simulink model "adcddcxaui_100"  (Simulink 6.2)
settings: Solver=ode45  StartTime=0.0  StopTime=1000  RelTol=1e-3
undefined symbols (not defined in the file): BitWidth
libraries: xbsIndex_r3 x358, casper_library x26, xps_library x12
(part 1 of 4)
settings Model: LastModifiedBy=lspitler
settings DebuggingCC: SolverPrmCheckMsg=warning

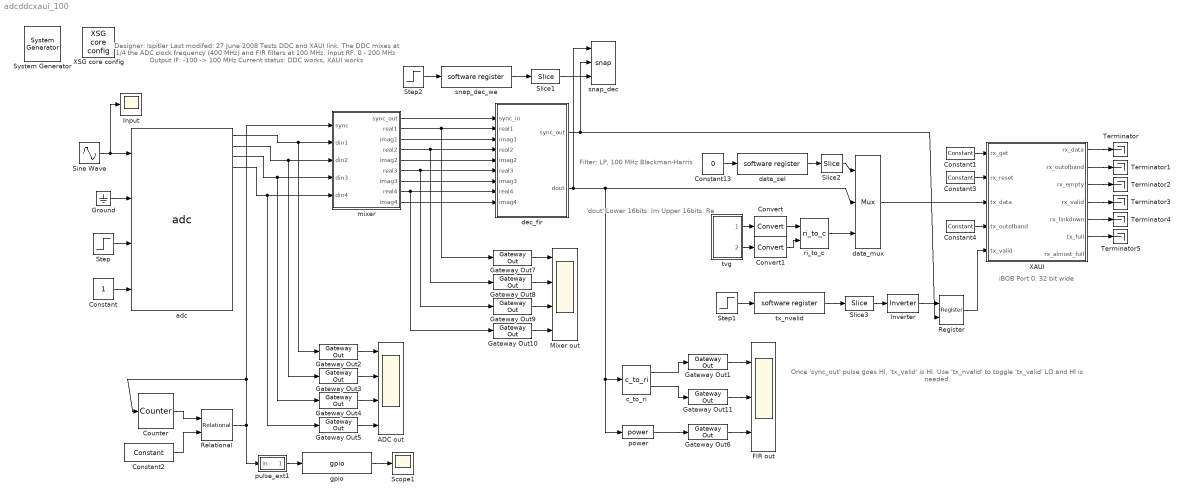
== system adcddcxaui_100 ==
  note: Designer: lspitler
      | Last modifed: 27 June 2008
      | Tests DDC and XAUI link.
      | The DDC mixes at 1/4 the ADC clock frequency (400 MHz)
      | and FIR filters at 100 MHz.
      | Input RF:  0 - 200 MHz
      | Output IF: -100 -> 100 MHz
      | Current status: DDC works, XAUI works
  note: Filter:
      | LP, 100 MHz Blackman-Harris
  note: 'dout'
      | Lower 16bits: Im
      | Upper 16bits: Re
  note: iBOB Port 0: 32 bit wide
  note: Once 'sync_out' pulse goes
      | HI, 'tx_valid' is HI.
      | Use 'tx_nvalid' to toggle
      | 'tx_valid' LO and HI is needed.
  " System Generator" : xbsIndex_r3/ System Generator  Tag=genX  xilinxfamily=Virtex2P  part=xc2vp50  speed=-7  package=ff1152  synthesis_tool=XST  directory=./adcddcxaui/sysgen  testbench=off  simulink_period=1  sysclk_period=5  incr_netlist=off  trim_vbits=Everywhere in SubSystem  dbl_ovrd=According to Block Masks  core_generation=According to Block Masks  run_coregen=off  deprecated_control=off  eval_field=0
      settings: AttributesFormatString=System\nGenerator
  ADC out : Scope  NumInputPorts=4
      settings: YMin=-5~-5~-5~-5  YMax=5~5~5~5  SaveName=ScopeData3
  Constant : Constant
  Constant1 : xbsIndex_r3/Constant  const=1  equ=P=C  arith_type=Boolean  n_bits=1  bin_pt=0  opselect=C  inp2=PCIN>>17  opr=+  inp1=P  carry=CIN  iostate=0  explicit_period=on  period=1  dbl_ovrd=off
  Constant13 : Constant  Value=0
  Constant2 : xbsIndex_r3/Constant  const=2^28-1  equ=P=C  arith_type=Unsigned  n_bits=32  bin_pt=0  opselect=C  inp2=PCIN>>17  opr=+  inp1=P  carry=CIN  iostate=0  explicit_period=on  period=1  dbl_ovrd=off
  Constant3 : xbsIndex_r3/Constant  const=0  equ=P=C  arith_type=Boolean  n_bits=1  bin_pt=0  opselect=C  inp2=PCIN>>17  opr=+  inp1=P  carry=CIN  iostate=0  explicit_period=on  period=1  dbl_ovrd=off
  Constant4 : xbsIndex_r3/Constant  const=0  equ=P=C  arith_type=Unsigned  n_bits=4  bin_pt=0  opselect=C  inp2=PCIN>>17  opr=+  inp1=P  carry=CIN  iostate=0  explicit_period=on  period=1  dbl_ovrd=off
  Convert : xbsIndex_r3/Convert  arith_type="Signed  (2's comp)"  n_bits=16  bin_pt=15  quantization=Truncate  overflow=Wrap  latency=0  explicit_period=on  period=1  dbl_ovrd=off  show_param=off  inserted_by_tool=off  pipeline=off
      settings: xl_area=[0, 0, 0, 0, 0, 0, 0]
  Convert1 : xbsIndex_r3/Convert  arith_type="Signed  (2's comp)"  n_bits=16  bin_pt=15  quantization=Truncate  overflow=Wrap  latency=0  explicit_period=on  period=1  dbl_ovrd=off  show_param=off  inserted_by_tool=off  pipeline=off
      settings: xl_area=[0, 0, 0, 0, 0, 0, 0]
  Counter : xbsIndex_r3/Counter  cnt_type=Free Running  n_bits=32  bin_pt=0  arith_type=Unsigned  start_count=0  cnt_to=Inf  cnt_by_val=1  operation=Up  explicit_period=on  period=1  load_pin=off  rst=on  en=off  dbl_ovrd=off  show_param=off  use_rpm=on  gen_core=off
      settings: xl_area=[0, 0, 0, 0, 0, 0, 0]
  FIR out : Scope  NumInputPorts=3
      settings: YMin=-5~-5~-5  YMax=5~5~5
  Gateway Out{1..11} (11 alike) : xbsIndex_r3/Gateway Out  output_type=Double  nbits=8  bin_pt=6  arith_type=Boolean  quantization=Truncate  overflow=Wrap  hdl_port=on  timing_constraint=None  locs_specified=off  LOCs={}  needs_fixed_name=off  show_param=off
      settings: xl_area=[0, 0, 0, 0, 0, 0, 0]
  Ground : Ground
  Input : Scope
      settings: SaveName=ScopeData2
  Inverter : xbsIndex_r3/Inverter  latency=0  explicit_period=on  period=1  en=off  dbl_ovrd=off  show_param=off
      settings: xl_area=[0, 0, 0, 0, 0, 0, 0]
  Mixer out : Scope  NumInputPorts=4
      settings: YMin=-5~-5~-5~-5  YMax=5~5~5~5  SaveName=ScopeData4
  Register : xbsIndex_r3/Register  init=0  reg_only_valid=off  explicit_period=on  period=1  rst=off  en=on  out_en=off  dbl_ovrd=off  show_param=off
      settings: xl_area=[0, 0, 0, 0, 0, 0, 0]
  Relational : xbsIndex_r3/Relational  mode=a=b  latency=0  explicit_period=on  period=1  en=off  dbl_ovrd=off  show_param=off
      settings: xl_area=[0, 0, 0, 0, 0, 0, 0]
  Scope1 : Scope
      settings: SaveName=ScopeData5
  Sine Wave : Sin  Frequency=100e6/(2*pi)  SampleTime=0.25
  Slice1 : xbsIndex_r3/Slice  mode=Lower Bit Location + Width  nbits=1  bit1=0  base1=MSB of Input  bit0=0  base0=LSB of Input  boolean_output=on  explicit_period=off  period=1  dbl_ovrd=off
  Slice2 : xbsIndex_r3/Slice  mode=Lower Bit Location + Width  nbits=1  bit1=0  base1=MSB of Input  bit0=0  base0=LSB of Input  boolean_output=off  explicit_period=off  period=1  dbl_ovrd=off
  Slice3 : xbsIndex_r3/Slice  mode=Lower Bit Location + Width  nbits=1  bit1=0  base1=MSB of Input  bit0=0  base0=LSB of Input  boolean_output=on  explicit_period=off  period=1  dbl_ovrd=off
  Step : Step  SampleTime=0
  Step1 : Step  SampleTime=0
  Step2 : Step  SampleTime=0
  Terminator{,1..5} (6 alike) : Terminator
  XAUI : Subsystem  Tag=xps:xaui  AncestorBlock=xps_library/XAUI  mask(xaui){demux=2, port=iBOB:0, show_param=off, pre_emph=3, swing=800}
      mask prompts: show_param "---------------------- Show Implementation Parameters -----------------------------------------------------------------------------------"; pre_emph "Pre-emphasis"; swing "Differential swing"
      mask help: XAUI block for sending and receiving point-to-point, streaming data over the BEE2 and iBOB's CX4 connectors. NOTE: A new version of this block is in development.
      mask init:
      | xaui_mask;
      mask Help: eval('xlWeb([getenv(''MLIB_ROOT''), ''\doc\html\com_xaui\com_xaui.html''])')
      mask StyleString: popup(1|2),popup(iBOB:0|iBOB:1|BEE2_ctrl:0|BEE2_ctrl:1|BEE2_usr:0|BEE2_usr:1|BEE2_usr:2|BEE2_usr:3|CORR:0),checkbox,popup(0|1|2|3),popup(400|500|600|700|800)
      mask CallbackString:
      | ||myname=gcb;
      | if strcmp(get_param(myname, 'show_param'), 'on')
      |     set_param(myname, 'MaskVisibilities', {'on','on','on','on','on'});
      | else
      |     set_param(myname, 'MaskVisibilities', {'on','on','on','off','off'});
      | end||
  XSG core config : xps_library/XSG core config  Tag=xps:xsg  hw_sys=iBOB  ibob_linux=off  clk_src=adc0_clk  gpio_clk_io_group=iBOB:sma  gpio_clk_bit_index=0  clk_rate=100  sample_period=1  synthesis_tool=XST  mpc_type=powerpc405
  adc : xps_library/adc  Tag=xps:adc  adc_brd=iBOB:adc0  adc_clk_rate=400  adc_interleave=off  sample_period=1
  c_to_ri : casper_library/Misc/c_to_ri  n_bits=16  bin_pt=15
      settings: AttributesFormatString=16_15 r/i
  data_mux : xbsIndex_r3/Mux  inputs=2  precision=Full  arith_type="Signed  (2's comp)"  n_bits=8  bin_pt=2  quantization=Truncate  overflow=Wrap  latency=0  explicit_period=on  period=1  en=off  dbl_ovrd=off  show_param=off  mux_type=off  use_rpm=off  gen_core=off
      settings: xl_area=[0, 0, 0, 0, 0, 0, 0]
  data_sel : xps_library/software register  Tag=xps:sw_reg  io_dir=From Processor  arith_type=Unsigned  bitwidth=32  bin_pt=0  sample_period=1  gw_name=adcddcxaui_100_data_sel_user_data_out
  dec_fir : Subsystem  AncestorBlock=casper_library/Downconverter/dec_fir  mask(dec_fir){n_inputs=4, coeff=[-2.32022704382012e-007 -1.96793901412143e-006 -6.75154059522534e-006 -6.84714551426329e-006 1.40951673085967e-005 6.32691079378998e-005 0.00010979324523175 7.49325945610502e-005 -0.000118431156085725 -0.000436437229681919 -0.000646606487019754 -0.00038661995841418 0.000545438664656682 0.00182028229313871 0.00247093665916482 0.00136692957063967 -0.00179924993407727 -0.00564405140037139 -0.00725034616519259 -0.00381996817794863 0.0048188087277704 0.014580065732477 0.0181905286238286 0.00938133540413822 -0.0116934149100173 -0.0353791342600711 -0.0448597099993105 -0.0240746309704666 0.0324249154639043 0.113465227678761 0.193526756592295 0.243273145290241 0.243273145290241 0.193526756592295 0.113465227678761 0.0324249154639043 -0.0240746309704666 -0.0448597099993105 -0.0353791342600711 -0.0116934149100173 0.00938133540413823 0.0181905286238286 0.014580065732477 0.0048188087277704 -0.00381996817794864 -0.00725034616519259 -0.00564405140037139 -0.00179924993407727 0.00136692957063967 0.00247093665916482 0.00182028229313871 0.000545438664656683 -0.00038661995841418 -0.000646606487019753 -0.00043643722968192 -0.000118431156085725 7.49325945610503e-005 0.00010979324523175 6.32691079379003e-005 1.40951673085965e-005 -6.84714551426338e-006 -6.75154059522503e-006 -1.96793901412178e-006 -2.32022704382012e-007], n_bits=16, quantization=Truncate, add_latency=2, mult_latency=2}
      mask prompts: n_inputs "Number of Parallel Streams"; coeff "Coefficients"; n_bits "Bit Width Out"; quantization "Quantization Behavior"; add_latency "Add Latency"; mult_latency "Mult Latency"
      mask help: FIR filter which can handle multiple time samples in parallel and decimates down to 1 time sample. If coefficients are symmetric, will automatically fold before multiplying.
      mask init:
      | dec_fir_init(gcb, ...
      |     'n_inputs', n_inputs, ...
      |     'coeff', coeff, ...
      |     'n_bits', n_bits, ...
      |     'quantization', quantization, ...
      |     'add_latency', add_latency, ...
      |     'mult_latency', mult_latency);
      settings: AttributesFormatString=|
      | 64 taps
      | 16_15 r/i
      mask Help:
      | <h1>Description</h1>
      | 
      | FIR filter which can handle multiple time samples in parallel and decimates down to 1 time sample.  If coefficients are symmetric, will automatically fold before multiplying.
      | 
      | <h2>Mask Parameters</h2>
      | 
      | <b>Number of Parallel Streams</b> (n_inputs): The number of time samples which arrive in parallel.<br><br>
      | 
      | <b>Coefficients</b> (coeff): The FIR coefficients.  If this vector is symmetric, the FIR will automatically fold before multiplying.<br><br>
      | 
      | <b>Bit Width Out</b> (n_bits): The number of bits in each real/imag sample of the complex number that is output.<br><br>
      | 
      | <b>Quantization Behavior</b> (quantization): The quantization behavior used in converting to the output bit width.<br><br>
      | 
      | 
      | <b>Add Latency</b> (add_latency) = The latency of adders/converters.<br><br>
      | 
      | <b>Mult Latency</b> (mult_latency) = The latency of multipliers.<br><br>
      mask StyleString: edit,edit,edit,popup(Truncate|Round  (unbiased: +/- Inf)|Round  (unbiased: Even Values)),edit,edit
  gpio : xps_library/gpio  Tag=xps:gpio  io_group=iBOB:led  io_dir=out  arith_type=Boolean  bitwidth=1  bin_pt=0  bit_index=7  sample_period=1  use_single_ended=off  use_ddr=off  reg_iob=off  reg_clk_phase=0  termination=None
  mixer : Subsystem  AncestorBlock=casper_library/Downconverter/mixer  mask(mixer){freq_div=4, freq=1, nstreams=4, n_bits=8, bram_latency=2, mult_latency=3}
      mask prompts: freq_div "Frequency Divisions (M)"; freq "Mixing Frequency (? / M*2pi)"; nstreams "Number of Parallel Streams"; n_bits "Bit Width"; bram_latency "BRAM Latency"; mult_latency "Mult Latency"
      mask help: Digitally mixes an input signal (which can be several samples in parallel) with an LO of the indicated frequency (which is some fraction of the native FPGA clock rate).
      mask init:
      | mixer_init(gcb, ...
      |     'freq_div', freq_div, ...
      |     'freq', freq, ...
      |     'nstreams', nstreams, ...
      |     'n_bits', n_bits, ...
      |     'bram_latency', bram_latency, ...
      |     'mult_latency', mult_latency);
      settings: AttributesFormatString=lo at -1/4
      mask Help:
      | <h1>Description</h1>
      | 
      | Digitally mixes an input signal (which can be several samples in parallel) with an LO of the indicated frequency (which is some fraction of the native FPGA clock rate).
      | 
      | <h2>Mask Parameters</h2>
      | 
      | <b>Frequency Divisions</b> (freq_div):  The (power of 2) denominator of the mixing frequency. <br><br>
      | 
      | <b>Mixing Frequency</b> (freq) = The numerator of the mixing frequency.<br><br>
      | 
      | <b>Number of Parallel Streams</b> (nstreams) = The number of samples which arrive in parallel.<br><br>
      | 
      | <b>Bit Width</b> (n_bits) = The bitwidth of LO samples.<br><br>
      | 
      | <b>BRAM Latency</b> (bram_latency) = The latency of sine/cos lookup table.<br><br>
      | 
      | <b>MULT Latency</b> (mult_latency) = The latency of mixing multipliers.<br><br>
      | 
      | <h2> Usage </h2>
      | M = Frequency Divisions<br>
      | F = Mixing Frequency<br>
      | M and F must both be integers, and M must be a power of 2. The ratio F/M should equal the ratio f/r where r is the data rate of the sampled signal. For example, an F/M of 3/16 would downmix an 800Msps signal with an LO of 150MHz.
  power : casper_library/Misc/power  BitWidth=32
  pulse_ext1 : Subsystem  mask{pulse_len=2^23}
      mask prompts: pulse_len "Length of Pulse"
      mask init:
      | bits = ceil(log2(pulse_len+1));
  ri_to_c : casper_library/Misc/ri_to_c
  snap_dec : casper_library/Scopes/snap  nsamples=11
  snap_dec_we : xps_library/software register  Tag=xps:sw_reg  io_dir=From Processor  arith_type=Unsigned  bitwidth=32  bin_pt=0  sample_period=1  gw_name=adcddcxaui_100_snap_dec_we_user_data_out
  tvg : Subsystem
  tx_nvalid : xps_library/software register  Tag=xps:sw_reg  io_dir=From Processor  arith_type=Unsigned  bitwidth=32  bin_pt=0  sample_period=1  gw_name=adcddcxaui_100_tx_nvalid_user_data_out
  wires:
  mixer/1(sync_out) -> dec_fir/1(sync_in)
  mixer/2(real1) -> Gateway Out7/1, dec_fir/2(real1)
  mixer/3(imag1) -> dec_fir/3(imag1)
  mixer/4(real2) -> Gateway Out8/1, dec_fir/4(real2)
  mixer/5(imag2) -> dec_fir/5(imag2)
  mixer/6(real3) -> Gateway Out9/1, dec_fir/6(real3)
  mixer/7(imag3) -> dec_fir/7(imag3)
  mixer/8(real4) -> Gateway Out10/1, dec_fir/8(real4)
  mixer/9(imag4) -> dec_fir/9(imag4)
  dec_fir/2(dout) -> snap_dec/1, power/1, c_to_ri/1, data_mux/2
  Constant1/1 -> XAUI/1(rx_get)
  Constant3/1 -> XAUI/2(rx_reset)
  Constant4/1 -> XAUI/4(tx_outofband)
  Gateway Out1/1 -> FIR out/1
  c_to_ri/1 -> Gateway Out1/1
  Gateway Out2/1 -> ADC out/1
  Gateway Out3/1 -> ADC out/2
  Gateway Out4/1 -> ADC out/3
  Gateway Out5/1 -> ADC out/4
  Gateway Out7/1 -> Mixer out/1
  Gateway Out8/1 -> Mixer out/2
  Gateway Out9/1 -> Mixer out/3
  Gateway Out10/1 -> Mixer out/4
  Gateway Out6/1 -> FIR out/3
  c_to_ri/2 -> Gateway Out11/1
  Gateway Out11/1 -> FIR out/2
  power/1 -> Gateway Out6/1
  Sine Wave/1 -> adc/1, Input/1
  Ground/1 -> adc/2
  adc/1 -> Gateway Out2/1, mixer/2(din1)
  adc/2 -> Gateway Out3/1, mixer/3(din2)
  adc/3 -> Gateway Out4/1, mixer/4(din3)
  adc/4 -> Gateway Out5/1, mixer/5(din4)
  Step/1 -> adc/3
  Constant/1 -> adc/4
  Counter/1 -> Relational/1
  Constant2/1 -> Relational/2
  pulse_ext1/1(out) -> gpio/1
  gpio/1 -> Scope1/1
  dec_fir/1(sync_out) -> snap_dec/2, Register/2
  snap_dec_we/1 -> Slice1/1
  Step2/1 -> snap_dec_we/1
  Slice1/1 -> snap_dec/3
  XAUI/1(rx_data) -> Terminator/1
  XAUI/2(rx_outofband) -> Terminator1/1
  XAUI/3(rx_empty) -> Terminator2/1
  XAUI/4(rx_valid) -> Terminator3/1
  XAUI/5(rx_linkdown) -> Terminator4/1
  XAUI/6(tx_full) -> Terminator5/1
  data_mux/1 -> XAUI/3(tx_data)
  data_sel/1 -> Slice2/1
  Constant13/1 -> data_sel/1
  Slice2/1 -> data_mux/1
  tvg/1(re_out) -> Convert/1
  tvg/2(im_out) -> Convert1/1
  Convert/1 -> ri_to_c/1
  Convert1/1 -> ri_to_c/2
  ri_to_c/1 -> data_mux/3
  Step1/1 -> tx_nvalid/1
  tx_nvalid/1 -> Slice3/1
  Register/1 -> XAUI/5(tx_valid)
  Relational/1 -> pulse_ext1/1(in), mixer/1(sync), Counter/1
  Inverter/1 -> Register/1
  Slice3/1 -> Inverter/1

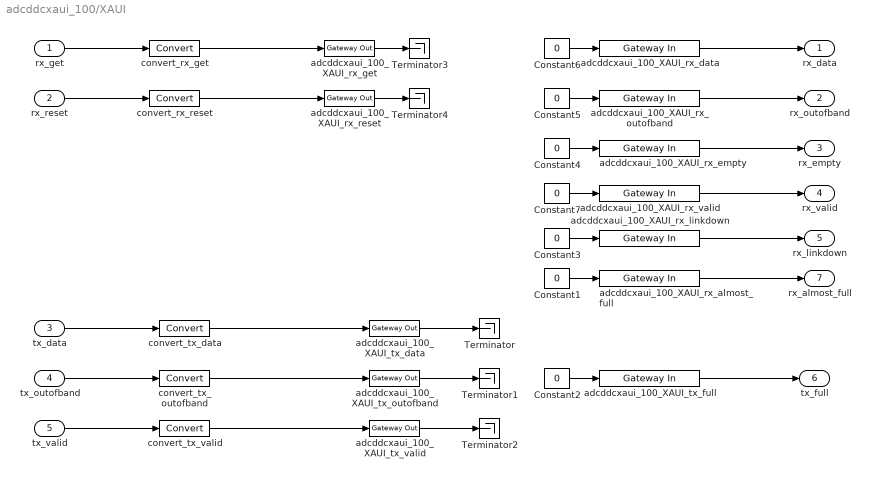
== system adcddcxaui_100/XAUI ==
  rx_get : Inport  Port=1  LatchInput=off
  rx_reset : Inport  Port=2  LatchInput=off
  tx_data : Inport  Port=3  LatchInput=off
  tx_outofband : Inport  Port=4  LatchInput=off
  tx_valid : Inport  Port=5  LatchInput=off
  Constant{1..7} (7 alike) : Constant  Value=0
  Terminator{,1..4} (5 alike) : Terminator
  adcddcxaui_100_XAUI_rx_almost_full : xbsIndex_r3/Gateway In  arith_type=Boolean  n_bits=1  bin_pt=0  quantization=Truncate  overflow=Wrap  period=1  timing_constraint=None  locs_specified=off  LOCs={}  needs_fixed_name=off  dbl_ovrd=off  show_param=off
      settings: xl_area=[0, 0, 0, 0, 0, 0, 0]
  adcddcxaui_100_XAUI_rx_data : xbsIndex_r3/Gateway In  arith_type=Unsigned  n_bits=32  bin_pt=0  quantization=Truncate  overflow=Wrap  period=1  timing_constraint=None  locs_specified=off  LOCs={}  needs_fixed_name=off  dbl_ovrd=off  show_param=off
      settings: xl_area=[0, 0, 0, 0, 0, 0, 0]
  adcddcxaui_100_XAUI_rx_empty : xbsIndex_r3/Gateway In  arith_type=Boolean  n_bits=1  bin_pt=0  quantization=Truncate  overflow=Wrap  period=1  timing_constraint=None  locs_specified=off  LOCs={}  needs_fixed_name=off  dbl_ovrd=off  show_param=off
      settings: xl_area=[0, 0, 0, 0, 0, 0, 0]
  adcddcxaui_100_XAUI_rx_get : xbsIndex_r3/Gateway Out  output_type=Double  nbits=8  bin_pt=6  arith_type=Boolean  quantization=Truncate  overflow=Wrap  hdl_port=on  timing_constraint=None  locs_specified=off  LOCs={}  needs_fixed_name=off  show_param=off
      settings: xl_area=[0, 0, 0, 0, 0, 0, 0]
  adcddcxaui_100_XAUI_rx_linkdown : xbsIndex_r3/Gateway In  arith_type=Boolean  n_bits=1  bin_pt=0  quantization=Truncate  overflow=Wrap  period=1  timing_constraint=None  locs_specified=off  LOCs={}  needs_fixed_name=off  dbl_ovrd=off  show_param=off
      settings: xl_area=[0, 0, 0, 0, 0, 0, 0]
  adcddcxaui_100_XAUI_rx_outofband : xbsIndex_r3/Gateway In  arith_type=Unsigned  n_bits=4  bin_pt=0  quantization=Truncate  overflow=Wrap  period=1  timing_constraint=None  locs_specified=off  LOCs={}  needs_fixed_name=off  dbl_ovrd=off  show_param=off
      settings: xl_area=[0, 0, 0, 0, 0, 0, 0]
  adcddcxaui_100_XAUI_rx_reset : xbsIndex_r3/Gateway Out  output_type=Double  nbits=8  bin_pt=6  arith_type=Boolean  quantization=Truncate  overflow=Wrap  hdl_port=on  timing_constraint=None  locs_specified=off  LOCs={}  needs_fixed_name=off  show_param=off
      settings: xl_area=[0, 0, 0, 0, 0, 0, 0]
  adcddcxaui_100_XAUI_rx_valid : xbsIndex_r3/Gateway In  arith_type=Boolean  n_bits=1  bin_pt=0  quantization=Truncate  overflow=Wrap  period=1  timing_constraint=None  locs_specified=off  LOCs={}  needs_fixed_name=off  dbl_ovrd=off  show_param=off
      settings: xl_area=[0, 0, 0, 0, 0, 0, 0]
  adcddcxaui_100_XAUI_tx_data : xbsIndex_r3/Gateway Out  output_type=Double  nbits=8  bin_pt=6  arith_type=Boolean  quantization=Truncate  overflow=Wrap  hdl_port=on  timing_constraint=None  locs_specified=off  LOCs={}  needs_fixed_name=off  show_param=off
      settings: xl_area=[0, 0, 0, 0, 0, 0, 0]
  adcddcxaui_100_XAUI_tx_full : xbsIndex_r3/Gateway In  arith_type=Boolean  n_bits=1  bin_pt=0  quantization=Truncate  overflow=Wrap  period=1  timing_constraint=None  locs_specified=off  LOCs={}  needs_fixed_name=off  dbl_ovrd=off  show_param=off
      settings: xl_area=[0, 0, 0, 0, 0, 0, 0]
  adcddcxaui_100_XAUI_tx_outofband : xbsIndex_r3/Gateway Out  output_type=Double  nbits=8  bin_pt=6  arith_type=Boolean  quantization=Truncate  overflow=Wrap  hdl_port=on  timing_constraint=None  locs_specified=off  LOCs={}  needs_fixed_name=off  show_param=off
      settings: xl_area=[0, 0, 0, 0, 0, 0, 0]
  adcddcxaui_100_XAUI_tx_valid : xbsIndex_r3/Gateway Out  output_type=Double  nbits=8  bin_pt=6  arith_type=Boolean  quantization=Truncate  overflow=Wrap  hdl_port=on  timing_constraint=None  locs_specified=off  LOCs={}  needs_fixed_name=off  show_param=off
      settings: xl_area=[0, 0, 0, 0, 0, 0, 0]
  convert_rx_get : xbsIndex_r3/Convert  arith_type=Boolean  n_bits=64  bin_pt=0  quantization=Truncate  overflow=Wrap  latency=0  explicit_period=off  period=1  dbl_ovrd=off  show_param=off  inserted_by_tool=off  pipeline=off
      settings: xl_area=[0, 0, 0, 0, 0, 0, 0]
  convert_rx_reset : xbsIndex_r3/Convert  arith_type=Boolean  n_bits=1  bin_pt=0  quantization=Truncate  overflow=Wrap  latency=0  explicit_period=off  period=1  dbl_ovrd=off  show_param=off  inserted_by_tool=off  pipeline=off
      settings: xl_area=[0, 0, 0, 0, 0, 0, 0]
  convert_tx_data : xbsIndex_r3/Convert  arith_type=Unsigned  n_bits=32  bin_pt=0  quantization=Truncate  overflow=Wrap  latency=0  explicit_period=off  period=1  dbl_ovrd=off  show_param=off  inserted_by_tool=off  pipeline=off
      settings: xl_area=[0, 0, 0, 0, 0, 0, 0]
  convert_tx_outofband : xbsIndex_r3/Convert  arith_type=Unsigned  n_bits=4  bin_pt=0  quantization=Truncate  overflow=Wrap  latency=0  explicit_period=off  period=1  dbl_ovrd=off  show_param=off  inserted_by_tool=off  pipeline=off
      settings: xl_area=[0, 0, 0, 0, 0, 0, 0]
  convert_tx_valid : xbsIndex_r3/Convert  arith_type=Boolean  n_bits=1  bin_pt=0  quantization=Truncate  overflow=Wrap  latency=0  explicit_period=off  period=1  dbl_ovrd=off  show_param=off  inserted_by_tool=off  pipeline=off
      settings: xl_area=[0, 0, 0, 0, 0, 0, 0]
  rx_data : Outport
  rx_outofband : Outport  Port=2
  rx_empty : Outport  Port=3
  rx_valid : Outport  Port=4
  rx_linkdown : Outport  Port=5
  tx_full : Outport  Port=6
  rx_almost_full : Outport  Port=7
  wires:
  Constant1/1 -> adcddcxaui_100_XAUI_rx_almost_full/1
  adcddcxaui_100_XAUI_rx_almost_full/1 -> rx_almost_full/1
  adcddcxaui_100_XAUI_rx_valid/1 -> rx_valid/1
  Constant7/1 -> adcddcxaui_100_XAUI_rx_valid/1
  adcddcxaui_100_XAUI_rx_reset/1 -> Terminator4/1
  adcddcxaui_100_XAUI_rx_get/1 -> Terminator3/1
  Constant6/1 -> adcddcxaui_100_XAUI_rx_data/1
  Constant5/1 -> adcddcxaui_100_XAUI_rx_outofband/1
  Constant4/1 -> adcddcxaui_100_XAUI_rx_empty/1
  Constant3/1 -> adcddcxaui_100_XAUI_rx_linkdown/1
  Constant2/1 -> adcddcxaui_100_XAUI_tx_full/1
  adcddcxaui_100_XAUI_tx_valid/1 -> Terminator2/1
  adcddcxaui_100_XAUI_tx_outofband/1 -> Terminator1/1
  adcddcxaui_100_XAUI_tx_data/1 -> Terminator/1
  adcddcxaui_100_XAUI_tx_full/1 -> tx_full/1
  convert_tx_valid/1 -> adcddcxaui_100_XAUI_tx_valid/1
  tx_valid/1 -> convert_tx_valid/1
  convert_tx_outofband/1 -> adcddcxaui_100_XAUI_tx_outofband/1
  tx_outofband/1 -> convert_tx_outofband/1
  convert_tx_data/1 -> adcddcxaui_100_XAUI_tx_data/1
  tx_data/1 -> convert_tx_data/1
  adcddcxaui_100_XAUI_rx_linkdown/1 -> rx_linkdown/1
  adcddcxaui_100_XAUI_rx_empty/1 -> rx_empty/1
  adcddcxaui_100_XAUI_rx_outofband/1 -> rx_outofband/1
  adcddcxaui_100_XAUI_rx_data/1 -> rx_data/1
  convert_rx_reset/1 -> adcddcxaui_100_XAUI_rx_reset/1
  rx_reset/1 -> convert_rx_reset/1
  convert_rx_get/1 -> adcddcxaui_100_XAUI_rx_get/1
  rx_get/1 -> convert_rx_get/1

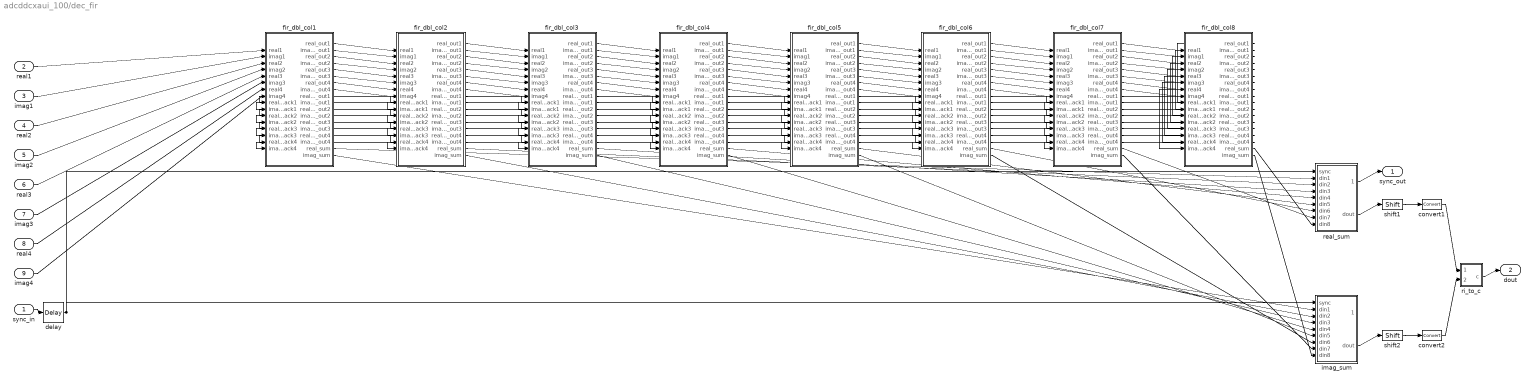
== system adcddcxaui_100/dec_fir ==
  sync_in : Inport  Port=1  LatchInput=off
  real1 : Inport  Port=2  LatchInput=off
  imag1 : Inport  Port=3  LatchInput=off
  real2 : Inport  Port=4  LatchInput=off
  imag2 : Inport  Port=5  LatchInput=off
  real3 : Inport  Port=6  LatchInput=off
  imag3 : Inport  Port=7  LatchInput=off
  real4 : Inport  Port=8  LatchInput=off
  imag4 : Inport  Port=9  LatchInput=off
  convert1 : xbsIndex_r3/Convert  arith_type="Signed  (2's comp)"  n_bits=16  bin_pt=15  quantization=Truncate  overflow=Saturate  latency=2  explicit_period=on  period=1  dbl_ovrd=off  show_param=on  inserted_by_tool=off  pipeline=on
      settings: xl_area=[0, 0, 0, 0, 0, 0, 0]
  convert2 : xbsIndex_r3/Convert  arith_type="Signed  (2's comp)"  n_bits=16  bin_pt=15  quantization=Truncate  overflow=Saturate  latency=2  explicit_period=on  period=1  dbl_ovrd=off  show_param=on  inserted_by_tool=off  pipeline=on
      settings: xl_area=[0, 0, 0, 0, 0, 0, 0]
  delay : xbsIndex_r3/Delay  latency=28  reg_retiming=off  explicit_period=off  period=1  en=off  accept_only_valid=off  init_zero=on  dbl_ovrd=off  show_param=off
      settings: xl_area=[0, 0, 0, 0, 0, 0, 0]
  fir_dbl_col1 : Subsystem  AncestorBlock=casper_library/Downconverter/fir_dbl_col  mask(fir_dbl_col){n_inputs=4, coeff=[-6.8471455143e-006 -6.7515405952e-006 -1.9679390141e-006 -2.320227044e-007], add_latency=2, mult_latency=2}
      mask prompts: n_inputs "Inputs"; coeff "Coefficients"; add_latency "Add latency"; mult_latency "Mult Latency"
      mask init:
      | fir_dbl_col_init(gcb, ...
      |     'n_inputs', n_inputs, ...
      |     'coeff', coeff, ...
      |     'mult_latency', mult_latency, ...
      |     'add_latency', add_latency);
  fir_dbl_col2 : Subsystem  AncestorBlock=casper_library/Downconverter/fir_dbl_col  mask(fir_dbl_col){n_inputs=4, coeff=[7.49325945611e-005 0.0001097932452318 6.32691079379e-005 1.40951673086e-005], add_latency=2, mult_latency=2}
      mask prompts: n_inputs "Inputs"; coeff "Coefficients"; add_latency "Add latency"; mult_latency "Mult Latency"
      mask init:
      | fir_dbl_col_init(gcb, ...
      |     'n_inputs', n_inputs, ...
      |     'coeff', coeff, ...
      |     'mult_latency', mult_latency, ...
      |     'add_latency', add_latency);
  fir_dbl_col3 : Subsystem  AncestorBlock=casper_library/Downconverter/fir_dbl_col  mask(fir_dbl_col){n_inputs=4, coeff=[-0.0003866199584142 -0.0006466064870198 -0.0004364372296819 -0.0001184311560857], add_latency=2, mult_latency=2}
      mask prompts: n_inputs "Inputs"; coeff "Coefficients"; add_latency "Add latency"; mult_latency "Mult Latency"
      mask init:
      | fir_dbl_col_init(gcb, ...
      |     'n_inputs', n_inputs, ...
      |     'coeff', coeff, ...
      |     'mult_latency', mult_latency, ...
      |     'add_latency', add_latency);
  fir_dbl_col4 : Subsystem  AncestorBlock=casper_library/Downconverter/fir_dbl_col  mask(fir_dbl_col){n_inputs=4, coeff=[0.0013669295706397 0.0024709366591648 0.0018202822931387 0.0005454386646567], add_latency=2, mult_latency=2}
      mask prompts: n_inputs "Inputs"; coeff "Coefficients"; add_latency "Add latency"; mult_latency "Mult Latency"
      mask init:
      | fir_dbl_col_init(gcb, ...
      |     'n_inputs', n_inputs, ...
      |     'coeff', coeff, ...
      |     'mult_latency', mult_latency, ...
      |     'add_latency', add_latency);
  fir_dbl_col5 : Subsystem  AncestorBlock=casper_library/Downconverter/fir_dbl_col  mask(fir_dbl_col){n_inputs=4, coeff=[-0.0038199681779486 -0.0072503461651926 -0.0056440514003714 -0.0017992499340773], add_latency=2, mult_latency=2}
      mask prompts: n_inputs "Inputs"; coeff "Coefficients"; add_latency "Add latency"; mult_latency "Mult Latency"
      mask init:
      | fir_dbl_col_init(gcb, ...
      |     'n_inputs', n_inputs, ...
      |     'coeff', coeff, ...
      |     'mult_latency', mult_latency, ...
      |     'add_latency', add_latency);
  fir_dbl_col6 : Subsystem  AncestorBlock=casper_library/Downconverter/fir_dbl_col  mask(fir_dbl_col){n_inputs=4, coeff=[0.0093813354041382 0.0181905286238286 0.014580065732477 0.0048188087277704], add_latency=2, mult_latency=2}
      mask prompts: n_inputs "Inputs"; coeff "Coefficients"; add_latency "Add latency"; mult_latency "Mult Latency"
      mask init:
      | fir_dbl_col_init(gcb, ...
      |     'n_inputs', n_inputs, ...
      |     'coeff', coeff, ...
      |     'mult_latency', mult_latency, ...
      |     'add_latency', add_latency);
  fir_dbl_col7 : Subsystem  AncestorBlock=casper_library/Downconverter/fir_dbl_col  mask(fir_dbl_col){n_inputs=4, coeff=[-0.0240746309704666 -0.0448597099993105 -0.0353791342600711 -0.0116934149100173], add_latency=2, mult_latency=2}
      mask prompts: n_inputs "Inputs"; coeff "Coefficients"; add_latency "Add latency"; mult_latency "Mult Latency"
      mask init:
      | fir_dbl_col_init(gcb, ...
      |     'n_inputs', n_inputs, ...
      |     'coeff', coeff, ...
      |     'mult_latency', mult_latency, ...
      |     'add_latency', add_latency);
  fir_dbl_col8 : Subsystem  AncestorBlock=casper_library/Downconverter/fir_dbl_col  mask(fir_dbl_col){n_inputs=4, coeff=[0.243273145290241 0.193526756592295 0.113465227678761 0.0324249154639043], add_latency=2, mult_latency=2}
      mask prompts: n_inputs "Inputs"; coeff "Coefficients"; add_latency "Add latency"; mult_latency "Mult Latency"
      mask init:
      | fir_dbl_col_init(gcb, ...
      |     'n_inputs', n_inputs, ...
      |     'coeff', coeff, ...
      |     'mult_latency', mult_latency, ...
      |     'add_latency', add_latency);
  imag_sum : Subsystem  AncestorBlock=casper_library/Misc/adder_tree  mask(adder_tree){n_inputs=8, latency=2}
      mask prompts: n_inputs "Number of Inputs"; latency "Add Latency"
      mask help: Sums all inputs using a tree of adds and delays.
      mask init:
      | adder_tree_init(gcb, ...
      |     'n_inputs', n_inputs, ...
      |     'latency', latency);
      settings: AttributesFormatString=latency 6
      mask Help: eval('xlWeb([getenv(''MLIB_ROOT''), ''\doc\html\sp_adder_tree\sp_adder_tree.html''])')
  real_sum : Subsystem  AncestorBlock=casper_library/Misc/adder_tree  mask(adder_tree){n_inputs=8, latency=2}
      mask prompts: n_inputs "Number of Inputs"; latency "Add Latency"
      mask help: Sums all inputs using a tree of adds and delays.
      mask init:
      | adder_tree_init(gcb, ...
      |     'n_inputs', n_inputs, ...
      |     'latency', latency);
      settings: AttributesFormatString=latency 6
      mask Help: eval('xlWeb([getenv(''MLIB_ROOT''), ''\doc\html\sp_adder_tree\sp_adder_tree.html''])')
  ri_to_c : Subsystem
  shift1 : xbsIndex_r3/Shift  shift_dir=Left  shift_bits=1  precision=Full  arith_type="Signed  (2's comp)"  n_bits=8  bin_pt=2  quantization=Truncate  overflow=Wrap  latency=0  explicit_period=off  period=1  en=off  dbl_ovrd=off  show_param=off
      settings: xl_area=[0, 0, 0, 0, 0, 0, 0]
  shift2 : xbsIndex_r3/Shift  shift_dir=Left  shift_bits=1  precision=Full  arith_type="Signed  (2's comp)"  n_bits=8  bin_pt=2  quantization=Truncate  overflow=Wrap  latency=0  explicit_period=off  period=1  en=off  dbl_ovrd=off  show_param=off
      settings: xl_area=[0, 0, 0, 0, 0, 0, 0]
  sync_out : Outport
  dout : Outport  Port=2
  wires:
  real1/1 -> fir_dbl_col1/1(real1)
  imag1/1 -> fir_dbl_col1/2(imag1)
  real2/1 -> fir_dbl_col1/3(real2)
  imag2/1 -> fir_dbl_col1/4(imag2)
  real3/1 -> fir_dbl_col1/5(real3)
  imag3/1 -> fir_dbl_col1/6(imag3)
  real4/1 -> fir_dbl_col1/7(real4)
  imag4/1 -> fir_dbl_col1/8(imag4)
  fir_dbl_col1/17(real_sum) -> real_sum/2(din1)
  fir_dbl_col1/18(imag_sum) -> imag_sum/2(din1)
  fir_dbl_col1/1(real_out1) -> fir_dbl_col2/1(real1)
  fir_dbl_col1/2(imag_out1) -> fir_dbl_col2/2(imag1)
  fir_dbl_col1/3(real_out2) -> fir_dbl_col2/3(real2)
  fir_dbl_col1/4(imag_out2) -> fir_dbl_col2/4(imag2)
  fir_dbl_col1/5(real_out3) -> fir_dbl_col2/5(real3)
  fir_dbl_col1/6(imag_out3) -> fir_dbl_col2/6(imag3)
  fir_dbl_col1/7(real_out4) -> fir_dbl_col2/7(real4)
  fir_dbl_col1/8(imag_out4) -> fir_dbl_col2/8(imag4)
  fir_dbl_col2/17(real_sum) -> real_sum/3(din2)
  fir_dbl_col2/18(imag_sum) -> imag_sum/3(din2)
  fir_dbl_col2/1(real_out1) -> fir_dbl_col3/1(real1)
  fir_dbl_col2/2(imag_out1) -> fir_dbl_col3/2(imag1)
  fir_dbl_col2/3(real_out2) -> fir_dbl_col3/3(real2)
  fir_dbl_col2/4(imag_out2) -> fir_dbl_col3/4(imag2)
  fir_dbl_col2/5(real_out3) -> fir_dbl_col3/5(real3)
  fir_dbl_col2/6(imag_out3) -> fir_dbl_col3/6(imag3)
  fir_dbl_col2/7(real_out4) -> fir_dbl_col3/7(real4)
  fir_dbl_col2/8(imag_out4) -> fir_dbl_col3/8(imag4)
  fir_dbl_col3/17(real_sum) -> real_sum/4(din3)
  fir_dbl_col3/18(imag_sum) -> imag_sum/4(din3)
  fir_dbl_col3/1(real_out1) -> fir_dbl_col4/1(real1)
  fir_dbl_col3/2(imag_out1) -> fir_dbl_col4/2(imag1)
  fir_dbl_col3/3(real_out2) -> fir_dbl_col4/3(real2)
  fir_dbl_col3/4(imag_out2) -> fir_dbl_col4/4(imag2)
  fir_dbl_col3/5(real_out3) -> fir_dbl_col4/5(real3)
  fir_dbl_col3/6(imag_out3) -> fir_dbl_col4/6(imag3)
  fir_dbl_col3/7(real_out4) -> fir_dbl_col4/7(real4)
  fir_dbl_col3/8(imag_out4) -> fir_dbl_col4/8(imag4)
  fir_dbl_col4/17(real_sum) -> real_sum/5(din4)
  fir_dbl_col4/18(imag_sum) -> imag_sum/5(din4)
  fir_dbl_col4/1(real_out1) -> fir_dbl_col5/1(real1)
  fir_dbl_col4/2(imag_out1) -> fir_dbl_col5/2(imag1)
  fir_dbl_col4/3(real_out2) -> fir_dbl_col5/3(real2)
  fir_dbl_col4/4(imag_out2) -> fir_dbl_col5/4(imag2)
  fir_dbl_col4/5(real_out3) -> fir_dbl_col5/5(real3)
  fir_dbl_col4/6(imag_out3) -> fir_dbl_col5/6(imag3)
  fir_dbl_col4/7(real_out4) -> fir_dbl_col5/7(real4)
  fir_dbl_col4/8(imag_out4) -> fir_dbl_col5/8(imag4)
  fir_dbl_col5/17(real_sum) -> real_sum/6(din5)
  fir_dbl_col5/18(imag_sum) -> imag_sum/6(din5)
  fir_dbl_col5/1(real_out1) -> fir_dbl_col6/1(real1)
  fir_dbl_col5/2(imag_out1) -> fir_dbl_col6/2(imag1)
  fir_dbl_col5/3(real_out2) -> fir_dbl_col6/3(real2)
  fir_dbl_col5/4(imag_out2) -> fir_dbl_col6/4(imag2)
  fir_dbl_col5/5(real_out3) -> fir_dbl_col6/5(real3)
  fir_dbl_col5/6(imag_out3) -> fir_dbl_col6/6(imag3)
  fir_dbl_col5/7(real_out4) -> fir_dbl_col6/7(real4)
  fir_dbl_col5/8(imag_out4) -> fir_dbl_col6/8(imag4)
  fir_dbl_col6/17(real_sum) -> real_sum/7(din6)
  fir_dbl_col6/18(imag_sum) -> imag_sum/7(din6)
  fir_dbl_col6/1(real_out1) -> fir_dbl_col7/1(real1)
  fir_dbl_col6/2(imag_out1) -> fir_dbl_col7/2(imag1)
  fir_dbl_col6/3(real_out2) -> fir_dbl_col7/3(real2)
  fir_dbl_col6/4(imag_out2) -> fir_dbl_col7/4(imag2)
  fir_dbl_col6/5(real_out3) -> fir_dbl_col7/5(real3)
  fir_dbl_col6/6(imag_out3) -> fir_dbl_col7/6(imag3)
  fir_dbl_col6/7(real_out4) -> fir_dbl_col7/7(real4)
  fir_dbl_col6/8(imag_out4) -> fir_dbl_col7/8(imag4)
  fir_dbl_col7/17(real_sum) -> real_sum/8(din7)
  fir_dbl_col7/18(imag_sum) -> imag_sum/8(din7)
  fir_dbl_col7/1(real_out1) -> fir_dbl_col8/1(real1)
  fir_dbl_col7/2(imag_out1) -> fir_dbl_col8/2(imag1)
  fir_dbl_col7/3(real_out2) -> fir_dbl_col8/3(real2)
  fir_dbl_col7/4(imag_out2) -> fir_dbl_col8/4(imag2)
  fir_dbl_col7/5(real_out3) -> fir_dbl_col8/5(real3)
  fir_dbl_col7/6(imag_out3) -> fir_dbl_col8/6(imag3)
  fir_dbl_col7/7(real_out4) -> fir_dbl_col8/7(real4)
  fir_dbl_col7/8(imag_out4) -> fir_dbl_col8/8(imag4)
  fir_dbl_col8/17(real_sum) -> real_sum/9(din8)
  fir_dbl_col8/18(imag_sum) -> imag_sum/9(din8)
  real_sum/2(dout) -> shift1/1
  imag_sum/2(dout) -> shift2/1
  shift1/1 -> convert1/1
  shift2/1 -> convert2/1
  convert1/1 -> ri_to_c/1(re)
  convert2/1 -> ri_to_c/2(im)
  ri_to_c/1(c) -> dout/1
  sync_in/1 -> delay/1
  delay/1 -> real_sum/1(sync), imag_sum/1(sync)
  real_sum/1(sync_out) -> sync_out/1
  fir_dbl_col2/9(real_back_out1) -> fir_dbl_col1/9(real_back1)
  fir_dbl_col2/10(imag_back_out1) -> fir_dbl_col1/10(imag_back1)
  fir_dbl_col2/11(real_back_out2) -> fir_dbl_col1/11(real_back2)
  fir_dbl_col2/12(imag_back_out2) -> fir_dbl_col1/12(imag_back2)
  fir_dbl_col2/13(real_back_out3) -> fir_dbl_col1/13(real_back3)
  fir_dbl_col2/14(imag_back_out3) -> fir_dbl_col1/14(imag_back3)
  fir_dbl_col2/15(real_back_out4) -> fir_dbl_col1/15(real_back4)
  fir_dbl_col2/16(imag_back_out4) -> fir_dbl_col1/16(imag_back4)
  fir_dbl_col3/9(real_back_out1) -> fir_dbl_col2/9(real_back1)
  fir_dbl_col3/10(imag_back_out1) -> fir_dbl_col2/10(imag_back1)
  fir_dbl_col3/11(real_back_out2) -> fir_dbl_col2/11(real_back2)
  fir_dbl_col3/12(imag_back_out2) -> fir_dbl_col2/12(imag_back2)
  fir_dbl_col3/13(real_back_out3) -> fir_dbl_col2/13(real_back3)
  fir_dbl_col3/14(imag_back_out3) -> fir_dbl_col2/14(imag_back3)
  fir_dbl_col3/15(real_back_out4) -> fir_dbl_col2/15(real_back4)
  fir_dbl_col3/16(imag_back_out4) -> fir_dbl_col2/16(imag_back4)
  fir_dbl_col4/9(real_back_out1) -> fir_dbl_col3/9(real_back1)
  fir_dbl_col4/10(imag_back_out1) -> fir_dbl_col3/10(imag_back1)
  fir_dbl_col4/11(real_back_out2) -> fir_dbl_col3/11(real_back2)
  fir_dbl_col4/12(imag_back_out2) -> fir_dbl_col3/12(imag_back2)
  fir_dbl_col4/13(real_back_out3) -> fir_dbl_col3/13(real_back3)
  fir_dbl_col4/14(imag_back_out3) -> fir_dbl_col3/14(imag_back3)
  fir_dbl_col4/15(real_back_out4) -> fir_dbl_col3/15(real_back4)
  fir_dbl_col4/16(imag_back_out4) -> fir_dbl_col3/16(imag_back4)
  fir_dbl_col5/9(real_back_out1) -> fir_dbl_col4/9(real_back1)
  fir_dbl_col5/10(imag_back_out1) -> fir_dbl_col4/10(imag_back1)
  fir_dbl_col5/11(real_back_out2) -> fir_dbl_col4/11(real_back2)
  fir_dbl_col5/12(imag_back_out2) -> fir_dbl_col4/12(imag_back2)
  fir_dbl_col5/13(real_back_out3) -> fir_dbl_col4/13(real_back3)
  fir_dbl_col5/14(imag_back_out3) -> fir_dbl_col4/14(imag_back3)
  fir_dbl_col5/15(real_back_out4) -> fir_dbl_col4/15(real_back4)
  fir_dbl_col5/16(imag_back_out4) -> fir_dbl_col4/16(imag_back4)
  fir_dbl_col6/9(real_back_out1) -> fir_dbl_col5/9(real_back1)
  fir_dbl_col6/10(imag_back_out1) -> fir_dbl_col5/10(imag_back1)
  fir_dbl_col6/11(real_back_out2) -> fir_dbl_col5/11(real_back2)
  fir_dbl_col6/12(imag_back_out2) -> fir_dbl_col5/12(imag_back2)
  fir_dbl_col6/13(real_back_out3) -> fir_dbl_col5/13(real_back3)
  fir_dbl_col6/14(imag_back_out3) -> fir_dbl_col5/14(imag_back3)
  fir_dbl_col6/15(real_back_out4) -> fir_dbl_col5/15(real_back4)
  fir_dbl_col6/16(imag_back_out4) -> fir_dbl_col5/16(imag_back4)
  fir_dbl_col7/9(real_back_out1) -> fir_dbl_col6/9(real_back1)
  fir_dbl_col7/10(imag_back_out1) -> fir_dbl_col6/10(imag_back1)
  fir_dbl_col7/11(real_back_out2) -> fir_dbl_col6/11(real_back2)
  fir_dbl_col7/12(imag_back_out2) -> fir_dbl_col6/12(imag_back2)
  fir_dbl_col7/13(real_back_out3) -> fir_dbl_col6/13(real_back3)
  fir_dbl_col7/14(imag_back_out3) -> fir_dbl_col6/14(imag_back3)
  fir_dbl_col7/15(real_back_out4) -> fir_dbl_col6/15(real_back4)
  fir_dbl_col7/16(imag_back_out4) -> fir_dbl_col6/16(imag_back4)
  fir_dbl_col8/9(real_back_out1) -> fir_dbl_col7/9(real_back1)
  fir_dbl_col8/10(imag_back_out1) -> fir_dbl_col7/10(imag_back1)
  fir_dbl_col8/11(real_back_out2) -> fir_dbl_col7/11(real_back2)
  fir_dbl_col8/12(imag_back_out2) -> fir_dbl_col7/12(imag_back2)
  fir_dbl_col8/13(real_back_out3) -> fir_dbl_col7/13(real_back3)
  fir_dbl_col8/14(imag_back_out3) -> fir_dbl_col7/14(imag_back3)
  fir_dbl_col8/15(real_back_out4) -> fir_dbl_col7/15(real_back4)
  fir_dbl_col8/16(imag_back_out4) -> fir_dbl_col7/16(imag_back4)
  fir_dbl_col8/1(real_out1) -> fir_dbl_col8/9(real_back1)
  fir_dbl_col8/2(imag_out1) -> fir_dbl_col8/10(imag_back1)
  fir_dbl_col8/3(real_out2) -> fir_dbl_col8/11(real_back2)
  fir_dbl_col8/4(imag_out2) -> fir_dbl_col8/12(imag_back2)
  fir_dbl_col8/5(real_out3) -> fir_dbl_col8/13(real_back3)
  fir_dbl_col8/6(imag_out3) -> fir_dbl_col8/14(imag_back3)
  fir_dbl_col8/7(real_out4) -> fir_dbl_col8/15(real_back4)
  fir_dbl_col8/8(imag_out4) -> fir_dbl_col8/16(imag_back4)

== system adcddcxaui_100/mixer ==
  sync : Inport  Port=1  LatchInput=off
  din1 : Inport  Port=2  LatchInput=off
  din2 : Inport  Port=3  LatchInput=off
  din3 : Inport  Port=4  LatchInput=off
  din4 : Inport  Port=5  LatchInput=off
  dds : Subsystem  AncestorBlock=casper_library/Downconverter/dds  mask(dds){freq_div=4, freq=1, num_lo=4, n_bits=8, latency=2}
      mask prompts: freq_div "Frequency divisions (M)"; freq "Frequency (? / M*2pi)"; num_lo "Parallel LOs"; n_bits "Bit Width"
      mask init:
      | dds_init(gcb, ...
      |     'freq_div', freq_div, ...
      |     'freq', freq, ...
      |     'num_lo', num_lo, ...
      |     'n_bits', n_bits, ...
      |     'latency', latency);
      settings: AttributesFormatString=lo at -1/4
  delay : xbsIndex_r3/Delay  latency=3  reg_retiming=off  explicit_period=off  period=1  en=off  accept_only_valid=off  init_zero=on  dbl_ovrd=off  show_param=off
      settings: xl_area=[0, 0, 0, 0, 0, 0, 0]
  rcmult1 : Subsystem  AncestorBlock=casper_library/Downconverter/rcmult  mask(rcmult){latency=3}
  rcmult2 : Subsystem  AncestorBlock=casper_library/Downconverter/rcmult  mask(rcmult){latency=3}
  rcmult3 : Subsystem  AncestorBlock=casper_library/Downconverter/rcmult  mask(rcmult){latency=3}
  rcmult4 : Subsystem  AncestorBlock=casper_library/Downconverter/rcmult  mask(rcmult){latency=3}
  sync_out : Outport
  real1 : Outport  Port=2
  imag1 : Outport  Port=3
  real2 : Outport  Port=4
  imag2 : Outport  Port=5
  real3 : Outport  Port=6
  imag3 : Outport  Port=7
  real4 : Outport  Port=8
  imag4 : Outport  Port=9
  wires:
  rcmult4/2(imag) -> imag4/1
  rcmult4/1(real) -> real4/1
  dds/8(cos3) -> rcmult4/3(cos)
  dds/7(sin3) -> rcmult4/2(sin)
  din4/1 -> rcmult4/1(d)
  rcmult3/2(imag) -> imag3/1
  rcmult3/1(real) -> real3/1
  dds/6(cos2) -> rcmult3/3(cos)
  dds/5(sin2) -> rcmult3/2(sin)
  din3/1 -> rcmult3/1(d)
  rcmult2/2(imag) -> imag2/1
  rcmult2/1(real) -> real2/1
  dds/4(cos1) -> rcmult2/3(cos)
  dds/3(sin1) -> rcmult2/2(sin)
  din2/1 -> rcmult2/1(d)
  rcmult1/2(imag) -> imag1/1
  rcmult1/1(real) -> real1/1
  dds/2(cos0) -> rcmult1/3(cos)
  dds/1(sin0) -> rcmult1/2(sin)
  din1/1 -> rcmult1/1(d)
  delay/1 -> sync_out/1
  sync/1 -> delay/1

== system adcddcxaui_100/pulse_ext1 ==
  in : Inport  Port=1  LatchInput=off
  Constant5 : xbsIndex_r3/Constant  const=pulse_len  equ=P=C  arith_type=Unsigned  n_bits=bits  bin_pt=0  opselect=C  inp2=PCIN>>17  opr=+  inp1=P  carry=CIN  iostate=0  explicit_period=off  period=1  dbl_ovrd=off
  Counter3 : xbsIndex_r3/Counter  cnt_type=Free Running  n_bits=bits  bin_pt=0  arith_type=Unsigned  start_count=0  cnt_to=1023  cnt_by_val=1  operation=Up  explicit_period=on  period=1  load_pin=off  rst=on  en=on  dbl_ovrd=off  show_param=off  use_rpm=on  gen_core=off
      settings: xl_area=[0, 0, 0, 0, 0, 0, 0]
  Relational5 : xbsIndex_r3/Relational  mode=a!=b  latency=0  explicit_period=off  period=1  en=off  dbl_ovrd=off  show_param=off
      settings: xl_area=[0, 0, 0, 0, 0, 0, 0]
  posedge : Subsystem  Tag=Rising Edge Detector
  out : Outport
  wires:
  Counter3/1 -> Relational5/1
  Constant5/1 -> Relational5/2
  Relational5/1 -> Counter3/2, out/1
  in/1 -> posedge/1(In)
  posedge/1(Out) -> Counter3/1

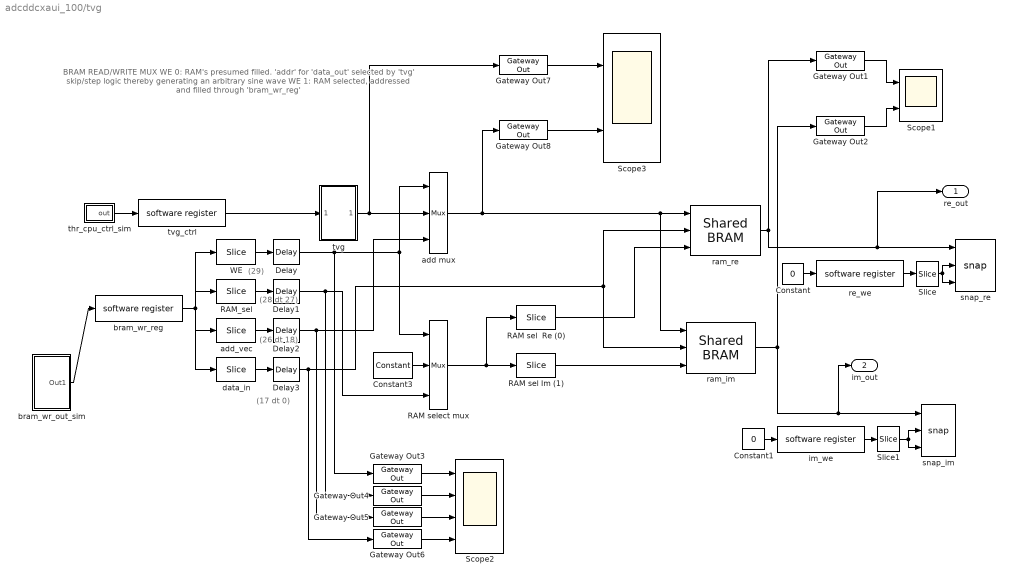
== system adcddcxaui_100/tvg ==
  note: (26 dt 18)
  note: (17 dt 0)
  note: (28 dt 27)
  note: (29)
  note: BRAM READ/WRITE MUX
      | WE 0: RAM's presumed filled.
      | 'addr' for 'data_out' selected
      | by 'tvg' skip/step logic thereby
      | generating an arbitrary sine wave
      | WE 1: RAM selected, addressed
      | and filled through
      | 'bram_wr_reg'
  Constant : Constant  Value=0
  Constant1 : Constant  Value=0
  Constant3 : xbsIndex_r3/Constant  const=0  equ=P=C  arith_type=Unsigned  n_bits=4  bin_pt=0  opselect=C  inp2=PCIN>>17  opr=+  inp1=P  carry=CIN  iostate=0  explicit_period=on  period=1  dbl_ovrd=off
  Delay{,1..3} (4 alike) : xbsIndex_r3/Delay  latency=1  reg_retiming=off  explicit_period=on  period=1  en=off  accept_only_valid=off  init_zero=on  dbl_ovrd=off  show_param=off
      settings: xl_area=[0, 0, 0, 0, 0, 0, 0]
  Gateway Out{1..8} (8 alike) : xbsIndex_r3/Gateway Out  output_type=Double  nbits=8  bin_pt=6  arith_type=Boolean  quantization=Truncate  overflow=Wrap  hdl_port=on  timing_constraint=None  locs_specified=off  LOCs={}  needs_fixed_name=off  show_param=off
      settings: xl_area=[0, 0, 0, 0, 0, 0, 0]
  RAM sel  Re (0) : xbsIndex_r3/Slice  mode=Lower Bit Location + Width  nbits=1  bit1=0  base1=MSB of Input  bit0=0  base0=LSB of Input  boolean_output=on  explicit_period=on  period=1  dbl_ovrd=off
  RAM sel Im (1) : xbsIndex_r3/Slice  mode=Lower Bit Location + Width  nbits=1  bit1=0  base1=MSB of Input  bit0=1  base0=LSB of Input  boolean_output=on  explicit_period=on  period=1  dbl_ovrd=off
  RAM select mux : xbsIndex_r3/Mux  inputs=2  precision=Full  arith_type="Signed  (2's comp)"  n_bits=8  bin_pt=2  quantization=Truncate  overflow=Wrap  latency=0  explicit_period=on  period=1  en=off  dbl_ovrd=off  show_param=off  mux_type=off  use_rpm=off  gen_core=off
      settings: xl_area=[0, 0, 0, 0, 0, 0, 0]
  RAM_sel : xbsIndex_r3/Slice  mode=Lower Bit Location + Width  nbits=2  bit1=10  base1=MSB of Input  bit0=27  base0=LSB of Input  boolean_output=off  explicit_period=on  period=1  dbl_ovrd=off
  Scope1 : Scope  NumInputPorts=2
      settings: YMin=-5~-5  YMax=5~5  SaveName=ScopeData2
  Scope2 : Scope  NumInputPorts=4
      settings: YMin=-5~-5~-5~-5  YMax=5~5~5~5
  Scope3 : Scope  NumInputPorts=2
      settings: YMin=-5~-5  YMax=5~5  SaveName=ScopeData3
  Slice : xbsIndex_r3/Slice  mode=Lower Bit Location + Width  nbits=1  bit1=0  base1=MSB of Input  bit0=0  base0=LSB of Input  boolean_output=on  explicit_period=off  period=1  dbl_ovrd=off
  Slice1 : xbsIndex_r3/Slice  mode=Lower Bit Location + Width  nbits=1  bit1=0  base1=MSB of Input  bit0=0  base0=LSB of Input  boolean_output=on  explicit_period=off  period=1  dbl_ovrd=off
  WE : xbsIndex_r3/Slice  mode=Lower Bit Location + Width  nbits=1  bit1=10  base1=MSB of Input  bit0=29  base0=LSB of Input  boolean_output=off  explicit_period=on  period=1  dbl_ovrd=off
  add mux : xbsIndex_r3/Mux  inputs=2  precision=Full  arith_type="Signed  (2's comp)"  n_bits=8  bin_pt=2  quantization=Truncate  overflow=Wrap  latency=0  explicit_period=on  period=1  en=off  dbl_ovrd=off  show_param=off  mux_type=off  use_rpm=off  gen_core=off
      settings: xl_area=[0, 0, 0, 0, 0, 0, 0]
  add_vec : xbsIndex_r3/Slice  mode=Lower Bit Location + Width  nbits=9  bit1=0  base1=MSB of Input  bit0=18  base0=LSB of Input  boolean_output=off  explicit_period=on  period=1  dbl_ovrd=off
  bram_wr_out_sim : Subsystem  mask{we_enable=0, ram_sel=3, add_vec=512, data_in=32}
      mask prompts: we_enable "Write enable"; ram_sel "RAM selector (1 = Re; 2 = Im; 3 = both)"; add_vec "RAM address"; data_in "Data in"
  bram_wr_reg : xps_library/software register  Tag=xps:sw_reg  io_dir=From Processor  arith_type=Unsigned  bitwidth=32  bin_pt=0  sample_period=1  gw_name=adcddcxaui_100_tvg_bram_wr_reg_user_data_out
  data_in : xbsIndex_r3/Slice  mode=Lower Bit Location + Width  nbits=18  bit1=0  base1=MSB of Input  bit0=0  base0=LSB of Input  boolean_output=off  explicit_period=on  period=1  dbl_ovrd=off
  im_we : xps_library/software register  Tag=xps:sw_reg  io_dir=From Processor  arith_type=Unsigned  bitwidth=32  bin_pt=0  sample_period=1  gw_name=adcddcxaui_100_tvg_im_we_user_data_out
  ram_im : xps_library/Shared BRAM  Tag=xps:bram  arith_type="Signed  (2's comp)"  addr_width=11  data_width=32  data_bin_pt=0  init_vals=[1:2^11]  sample_rate=1
  ram_re : xps_library/Shared BRAM  Tag=xps:bram  arith_type="Signed  (2's comp)"  addr_width=11  data_width=32  data_bin_pt=0  init_vals=[1:2^11]  sample_rate=1
  re_we : xps_library/software register  Tag=xps:sw_reg  io_dir=From Processor  arith_type=Unsigned  bitwidth=32  bin_pt=0  sample_period=1  gw_name=adcddcxaui_100_tvg_re_we_user_data_out
  snap_im : casper_library/Scopes/snap  nsamples=11
  snap_re : casper_library/Scopes/snap  nsamples=11
  thr_cpu_ctrl_sim : Subsystem  mask{tvg_skip=1, tvg_stall=2, tvg_length=5}
      mask prompts: tvg_skip "Skip"; tvg_stall "Stall"; tvg_length "Length"
      mask help:
      | Mux Data for CT and FFT Syncs:
      |
      | 0 -> Interchip Connection
      | 1 -> User Generated External Sync
      | 2 -> Periodic Sync Generator
      | 3 -> Periodic Sync Generator (Same as 2)
      |
      | Mux Data for CT and FFT Inputs:
      |
      | 0 -> Interchip Connection
      | 1 -> Test Vector Generator (TVG)
      | 2 -> All Zeroes (0's)
      | 3 -> All Ones (1's)
  tvg : Subsystem  mask(Test Vector Generator(TVG)){tvg_skip=1, tvg_stall=1, tvg_length=512}
      mask prompts: tvg_skip "Skip"; tvg_stall "Stall"; tvg_length "Length"
  tvg_ctrl : xps_library/software register  Tag=xps:sw_reg  io_dir=From Processor  arith_type=Unsigned  bitwidth=32  bin_pt=0  sample_period=1  gw_name=adcddcxaui_100_tvg_tvg_ctrl_user_data_out
  re_out : Outport
  im_out : Outport  Port=2
  wires:
  Constant1/1 -> im_we/1
  im_we/1 -> Slice1/1
  Slice1/1 -> snap_im/3, snap_im/2
  Constant/1 -> re_we/1
  re_we/1 -> Slice/1
  Slice/1 -> snap_re/3, snap_re/2
  Gateway Out8/1 -> Scope3/2
  Gateway Out7/1 -> Scope3/1
  Delay3/1 -> ram_im/2, ram_re/2, Gateway Out6/1
  Delay2/1 -> add mux/3, Gateway Out5/1
  Delay1/1 -> RAM select mux/3, Gateway Out4/1
  Delay/1 -> RAM select mux/1, add mux/1, Gateway Out3/1
  Gateway Out6/1 -> Scope2/4
  Gateway Out5/1 -> Scope2/3
  Gateway Out4/1 -> Scope2/2
  Gateway Out3/1 -> Scope2/1
  bram_wr_out_sim/1(Out1) -> bram_wr_reg/1
  ram_im/1 -> im_out/1, snap_im/1, Gateway Out2/1
  ram_re/1 -> re_out/1, snap_re/1, Gateway Out1/1
  RAM sel Im (1)/1 -> ram_im/3
  data_in/1 -> Delay3/1
  add mux/1 -> Gateway Out8/1, ram_re/1, ram_im/1
  RAM_sel/1 -> Delay1/1
  add_vec/1 -> Delay2/1
  bram_wr_reg/1 -> WE/1, RAM_sel/1, add_vec/1, data_in/1
  thr_cpu_ctrl_sim/1(out) -> tvg_ctrl/1
  Gateway Out2/1 -> Scope1/2
  Gateway Out1/1 -> Scope1/1
  WE/1 -> Delay/1
  RAM sel  Re (0)/1 -> ram_re/3
  RAM select mux/1 -> RAM sel Im (1)/1, RAM sel  Re (0)/1
  Constant3/1 -> RAM select mux/2
  tvg/1(Out1) -> Gateway Out7/1, add mux/2
  tvg_ctrl/1 -> tvg/1(In1)
